simulink model "saturatedFlipflop"  (R2018b)
settings: Solver=VariableStepAuto  StartTime=0.0  StopTime=Inf  RelTol=1e-3
settings Model: EnablePacing=on  Creator=Sjoerd  LastModifiedBy=Sjoerd

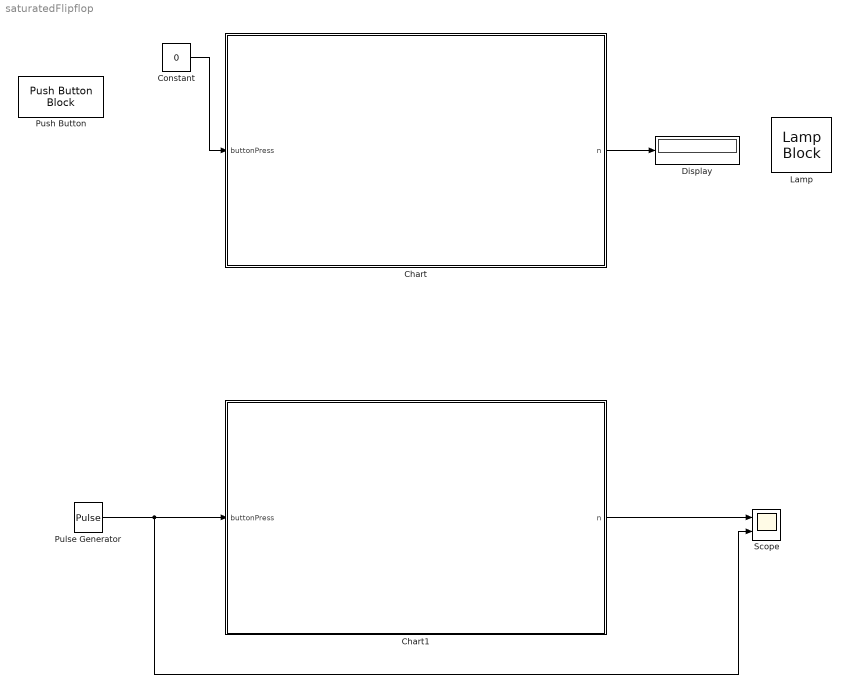
== system saturatedFlipflop ==
  Chart : Stateflow chart  TreatAsAtomicUnit=on
  Chart1 : Stateflow chart  TreatAsAtomicUnit=on
  Constant : Constant  Value=0
  Display : Display
  Lamp : LampBlock  WebBlockId=4
  Pulse Generator : DiscretePulseGenerator  PulseType=Time based  Period=5  PulseWidth=50  PhaseDelay=10
  Push Button : PushButtonBlock  WebBlockId=2
  Scope : Scope  NumInputPorts=2
  wires:
  Constant/1 -> Chart/1(buttonPress)
  Chart/1(n) -> Display/1
  Pulse Generator/1 -> Scope/2, Chart1/1(buttonPress)
  Chart1/1(n) -> Scope/1

== stateflow chart saturatedFlipflop/Chart1 ==
  state NotPressed1
  state Pressed1
  state NotPressed2
  state Pressed2
  state NotPressed3
  (default) -> NotPressed1 : {n = 0}
  NotPressed1 -> Pressed1 : [buttonPress == 1]{n = 1}
  Pressed1 -> NotPressed2 : [buttonPress == 0]
  NotPressed2 -> Pressed2 : [buttonPress == 1]{n = 2}
  Pressed2 -> NotPressed3 : [buttonPress == 0]
  NotPressed3 -> Pressed2 : [buttonPress == 1]
  data: buttonPress input; n output

== stateflow chart saturatedFlipflop/Chart ==
  state NotPressed1
  state Pressed1
  state NotPressed2
  state Pressed2
  state NotPressed3
  (default) -> NotPressed1 : {n = 0}
  NotPressed1 -> Pressed1 : [buttonPress == 1]{n = 1}
  Pressed1 -> NotPressed2 : [buttonPress == 0]
  NotPressed2 -> Pressed2 : [buttonPress == 1]{n = 2}
  Pressed2 -> NotPressed3 : [buttonPress == 0]
  NotPressed3 -> Pressed2 : [buttonPress == 1]
  data: buttonPress input; n output
